simulink model "Lagrange_og"  (R2017b)
settings: Solver=ode45  StartTime=0.0  StopTime=10  RelTol=1e-3  EnableMultiTasking=on
values from neighbouring files (symbols this model uses):
  parameters = [m1,m2,I1,I2,a1,a2,l1,l2,g]    [Lag_main.m]
  statei = [[0;0],[0;0],[0;0]]    [Lag_main.m]
undefined symbols (not defined in the file or in its folder): statef
settings Model: Creator=RIKEN  LastModifiedBy=minakata
settings DataIOCC: LimitDataPoints=on  SaveFormat=Array
settings OptimizationCC: ExpressionDepthLimit=2147483647  LifeSpan=inf
settings DebuggingCC: UnderspecifiedInitializationDetection=Classic  MergeDetectMultiDrivingBlocksExec=none  StateNameClashWarn=warning  SFUnexpectedBacktrackingDiag=warning  SFNoUnconditionalDefaultTransitionDiag=warning  SFExecutionAtInitializationDiag=none
settings HardwareCC: ProdBitPerPointer=32  ProdBitPerSizeT=32  ProdBitPerPtrDiffT=32  ProdLargestAtomicFloat=None  ProdIntDivRoundTo=Undefined  ProdEndianess=Unspecified  ProdWordSize=32  ProdHWDeviceType=32-bit Generic
settings ModelReferenceCC: PropagateSignalLabelsOutOfModel=off
settings CodeAppCC: StateflowObjectComments=on
settings GRTTargetCC: TargetLangStandard=C89/C90 (ANSI)  GeneratePreprocessorConditionals=Disable all
settings ConfigComp: CovMetricSettings=dw  CovHtmlReporting=on  CovSaveCumulativeToWorkspaceVar=on  CovSaveSingleToWorkspaceVar=on  CovExternalEMLEnable=off

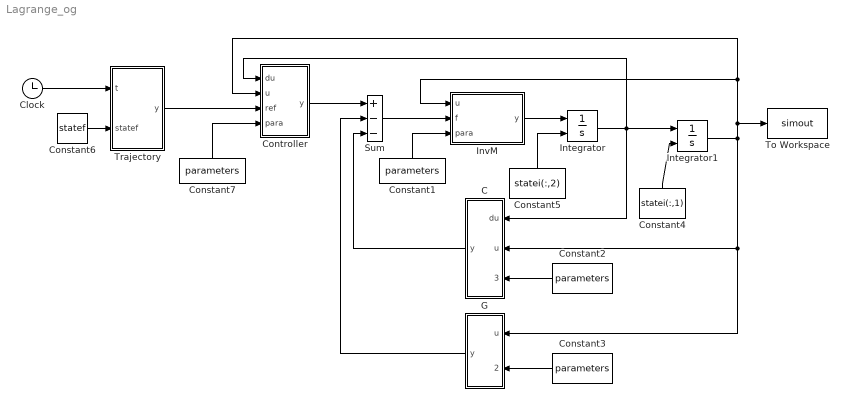
== system Lagrange_og ==
  C : MATLAB Function  TreatAsAtomicUnit=on
  Clock : Clock
  Constant{1..3,7} (4 alike) : Constant  Value=parameters
  Constant4 : Constant  Value=statei(:,1)
  Constant5 : Constant  Value=statei(:,2)
  Constant6 : Constant  Value=statef
  Controller : MATLAB Function  TreatAsAtomicUnit=on
  G : MATLAB Function  TreatAsAtomicUnit=on
  Integrator : Integrator  InitialConditionSource=external
  Integrator1 : Integrator  InitialConditionSource=external
  InvM : MATLAB Function  TreatAsAtomicUnit=on
  Sum : Sum  Inputs=+--
  To Workspace : ToWorkspace  VariableName=simout  SaveFormat=Timeseries  SampleTime=-1
  Trajectory : MATLAB Function  TreatAsAtomicUnit=on
  wires:
  Controller/1(y) -> Sum/1
  Sum/1 -> InvM/2(f)
  InvM/1(y) -> Integrator/1
  G/1(y) -> Sum/2
  C/1(y) -> Sum/3
  Constant1/1 -> InvM/3(para)
  Constant2/1 -> C/3(para)
  Constant3/1 -> G/2(para)
  Constant4/1 -> Integrator1/2
  Constant5/1 -> Integrator/2
  Constant7/1 -> Controller/4(para)
  Integrator1/1 -> To Workspace/1, Controller/2(u), InvM/1(u), G/1(u), C/2(u)
  Integrator/1 -> C/1(du), Controller/1(du), Integrator1/1
  Clock/1 -> Trajectory/1(t)
  Trajectory/1(y) -> Controller/3(ref)
  Constant6/1 -> Trajectory/2(statef)

== matlab function Lagrange_og/C ==
  data: du input; y output; u input; para input
function y = fcn(du,u,para)
%入力：各関節の回転速度
%      各関節の回転角度
%      システムに関するパラメータ
%出力：遠心力・コリオリ力
% C(theta,dtheta)
m2=para(2);
a1=para(5);
l2=para(8);
y1=-m2*a1*l2*sin(u(2))*(2*du(1)*du(2)+du(2)^2);
y2=m2*a1*l2*sin(u(2))*du(1)^2;
y = [y1;y2];

== matlab function Lagrange_og/InvM ==
  data: u input; f input; y output; para input
function y = fcn(u,f,para)
%入力：各関節の回転角度
%     トルク
%     システムに関するパラメータ
%出力：各関節の回転加速度
%Inverse M(theta)
m1=para(1);
m2=para(2);
I1=para(3);
I2=para(4);
a1=para(5);
l1=para(7);
l2=para(8);
g=para(9);
M11=I1+I2+m1*l1^2+m2*(a1^2+2*a1*l2*cos(u(2))+l2^2);
M12=I2+m2*(a1*l2*cos(u(2))+l2^2);
M21=M12;
M22=I2+m2*l2^2;
y = [M11,M12;M21,M22]\f;

== matlab function Lagrange_og/G ==
  data: u input; y output; para input
function y = fcn(u,para)
%入力：各関節の回転角度
%      システムに関するパラメータ
%出力：重力
% G(theta)
m1=para(1);
m2=para(2);
a1=para(5);
l1=para(7);
l2=para(8);
g=para(9);
y1=m1*g*l1*cos(u(1))+m2*g*(a1*cos(u(1))+l2*cos(u(1)+u(2)));
y2=m2*g*l2*cos(u(1)+u(2));
y = [y1;y2];

== matlab function Lagrange_og/Trajectory ==
  data: t input; statef input; y output
function y = fcn(t,statef)
%入力：時間t
%　　　目標状態statef
%出力：軌道
%５次関数を用いて軌道生成
%５次関数
%      f(0)=0;    f(T)=fy;
%     df(0)=0;   df(T)=0;
%    ddf(0)=0;  ddf(T)=0;
%    f=paraA1*t^5+paraA2*t^4+paraA3*t^3
T=10; %動く時間
%５次関数の係数
paraA=[T^5 T^4 T^3;...
    5*T^4 4*T^3 3*T^2;...
    20*T^3 12*T^2 6*T]\statef';
%軌道（各関節の参照回転角度）
tmp=[t^5 t^4 t^3;...
    5*t^4 4*t^3 3*t^2;...
    20*t^3 12*t^2 6*t]*paraA;
y = tmp';

== matlab function Lagrange_og/Controller ==
  data: du input; u input; y output; ref input; para input
function y = fcn(du,u,ref,para)
%入力：各関節の回転速度
%      各関節の回転角度
%      各関節の参照回転角度
%      システムに関するパラメータ
%出力：トルク
m1=para(1);
m2=para(2);
I1=para(3);
I2=para(4);
a1=para(5);
l1=para(7);
l2=para(8);
g=para(9);

D=100*eye(2);  %微分制御のゲイン
K=100*eye(2);  %比例制御のゲイン

%D=10*eye(2);  %微分制御のゲイン
%K=10*eye(2);  %比例制御のゲイン

%慣性力の係数
M11=I1+I2+m1*l1^2+m2*(a1^2+2*a1*l2*cos(u(2))+l2^2);
M12=I2+m2*(a1*l2*cos(u(2))+l2^2);
M21=M12;
M22=I2+m2*l2^2;
qref2dot=ref(:,3); %参照回転加速度
qrefdot=ref(:,2);  %参照回転速度
qref=ref(:,1);     %参照回転角度
%遠心力・コリオリ力
C1=-m2*a1*l2*sin(u(2))*(2*du(1)*du(2)+du(2)^2);
C2=m2*a1*l2*sin(u(2))*du(1)^2;
%重力
G1=m1*g*l1*cos(u(1))+m2*g*(a1*cos(u(1))+l2*cos(u(1)+u(2)));
G2=m2*g*l2*cos(u(1)+u(2));
y = [C1;C2]+[G1;G2]+...
    [M11,M12;M21,M22]*(qref2dot+D*(qrefdot-du)+K*(qref-u));
%y = [M11,M12;M21,M22]*(qref2dot+D*(qrefdot-du)+K*(qref-u));
